simulink model "aircraftControl_smallerStateEKF"  (R2014a)
settings: Solver=ode3  StartTime=0.0  StopTime=50  FixedStep=0.005  RelTol=1e-3
InitFcn:
  | InitialiseModel
values from neighbouring files (symbols this model uses):
  y0 = [0;0;-100;50;0;0;0;x(1);0;0;0;0]    [InitialiseModel.m]
settings Model: Creator=Rudaba  LastModifiedBy=Rudaba
settings DebuggingCC: FcnCallInpInsideContextMsg=EnableAllAsWarning

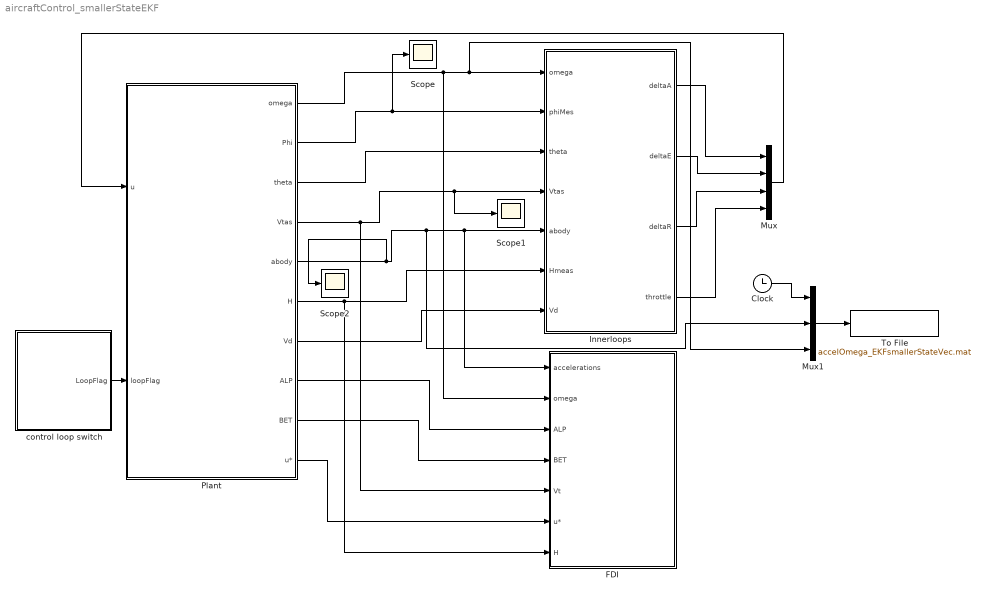
== system aircraftControl_smallerStateEKF ==
  Clock : Clock
  FDI : Subsystem
  Innerloops : Subsystem
  Mux : Mux
  Mux1 : Mux  Inputs=3
  Plant : Subsystem
  Scope : Scope
  Scope1 : Scope
  Scope2 : Scope
      settings: SaveName=ScopeData3
  To File : ToFile  Filename=accelOmega_EKFsmallerStateVec.mat  MatrixName=AO  SaveFormat=Timeseries
  control loop switch : Subsystem
  wires:
  Innerloops/2(deltaE) -> Mux/2
  Innerloops/1(deltaA) -> Mux/1
  Innerloops/3(deltaR) -> Mux/3
  control loop switch/1(LoopFlag) -> Plant/2(loopFlag)
  Innerloops/4(throttle) -> Mux/4
  Mux/1 -> Plant/1(u)
  Plant/1(omega) -> FDI/2(omega), Mux1/3, Innerloops/1(omega)
  Plant/2(Phi) -> Scope/1, Innerloops/2(phiMes)
  Plant/3(theta) -> Innerloops/3(theta)
  Plant/4(Vtas) -> FDI/5(Vt), Scope1/1, Innerloops/4(Vtas)
  Plant/5(abody) -> Scope2/1, Mux1/2, FDI/1(accelerations), Innerloops/5(abody)
  Plant/6(H) -> FDI/7(H), Innerloops/6(Hmeas)
  Plant/7(Vd) -> Innerloops/7(Vd)
  Plant/8(ALP) -> FDI/3(ALP)
  Plant/9(BET) -> FDI/4(BET)
  Plant/10(u*) -> FDI/6(u*)
  Clock/1 -> Mux1/1
  Mux1/1 -> To File/1

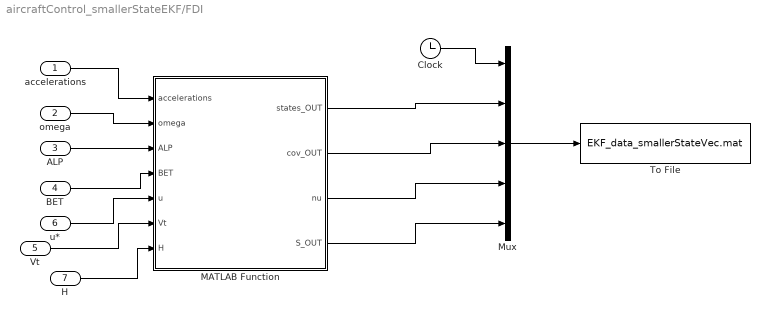
== system aircraftControl_smallerStateEKF/FDI ==
  accelerations : Inport
  omega : Inport  Port=2
  ALP : Inport  Port=3
  BET : Inport  Port=4
  Vt : Inport  Port=5
  u* : Inport  Port=6
  H : Inport  Port=7
  Clock : Clock
  MATLAB Function : MATLAB Function  TreatAsAtomicUnit=on
  Mux : Mux  Inputs=5
  To File : ToFile  Filename=EKF_data_smallerStateVec.mat  MatrixName=EKF  SaveFormat=Timeseries
  wires:
  MATLAB Function/1(states_OUT) -> Mux/2
  MATLAB Function/2(cov_OUT) -> Mux/3
  Mux/1 -> To File/1
  Clock/1 -> Mux/1
  accelerations/1 -> MATLAB Function/1(accelerations)
  omega/1 -> MATLAB Function/2(omega)
  ALP/1 -> MATLAB Function/3(ALP)
  BET/1 -> MATLAB Function/4(BET)
  u*/1 -> MATLAB Function/5(u)
  Vt/1 -> MATLAB Function/6(Vt)
  H/1 -> MATLAB Function/7(H)
  MATLAB Function/3(nu) -> Mux/4
  MATLAB Function/4(S_OUT) -> Mux/5

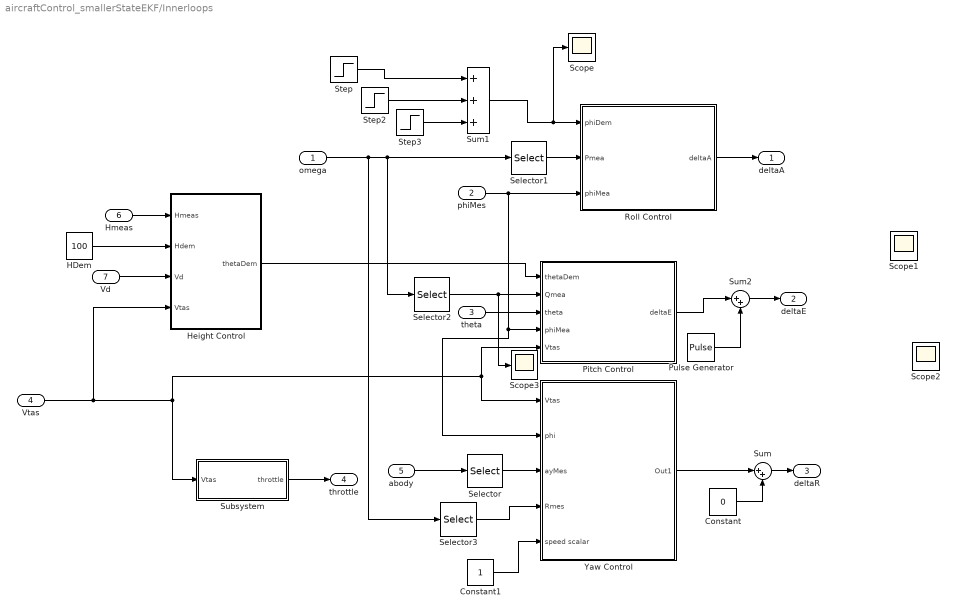
== system aircraftControl_smallerStateEKF/Innerloops ==
  omega : Inport
  phiMes : Inport  Port=2
  theta : Inport  Port=3
  Vtas : Inport  Port=4
  abody : Inport  Port=5
  Hmeas : Inport  Port=6
  Vd : Inport  Port=7
  Constant : Constant  Value=0
  Constant1 : Constant
  HDem : Constant  Value=100
  Height Control : Subsystem
  Pitch Control : Subsystem
  Pulse Generator : DiscretePulseGenerator  PulseType=Time based  Amplitude=0.1  Period=1  PulseWidth=50
  Roll Control : Subsystem
  Scope{,1..3} (4 alike) : Scope
      Scope settings: SaveName=ScopeData2
      Scope1 settings: SaveName=ScopeData11
      Scope2 settings: SaveName=ScopeData12
      Scope3 settings: SaveName=ScopeData13
  Selector : Selector  InputPortWidth=3  Indices=2
  Selector1 : Selector  InputPortWidth=3
  Selector2 : Selector  InputPortWidth=3  Indices=2
  Selector3 : Selector  InputPortWidth=3  Indices=3
  Step : Step  After=0.5  SampleTime=0
  Step2 : Step  Time=40  After=-1  SampleTime=0
  Step3 : Step  Time=70  After=0.5  SampleTime=0
  Subsystem : Subsystem
  Sum : Sum  Inputs=|++
  Sum1 : Sum  Inputs=+++
  Sum2 : Sum  Inputs=|++
  Yaw Control : Subsystem
  deltaA : Outport
  deltaE : Outport  Port=2
  deltaR : Outport  Port=3
  throttle : Outport  Port=4
  wires:
  Height Control/1(thetaDem) -> Pitch Control/1(thetaDem)
  omega/1 -> Selector3/1, Selector1/1, Selector2/1
  phiMes/1 -> Yaw Control/2(phi), Pitch Control/4(phiMea), Roll Control/3(phiMea)
  Selector2/1 -> Scope3/1, Pitch Control/2(Qmea)
  theta/1 -> Pitch Control/3(theta)
  Roll Control/1(deltaA) -> deltaA/1
  Yaw Control/1(Out1) -> Sum/1
  Constant1/1 -> Yaw Control/5(speed scalar)
  abody/1 -> Selector/1
  Selector/1 -> Yaw Control/3(ayMes)
  Constant/1 -> Sum/2
  Sum/1 -> deltaR/1
  Step/1 -> Sum1/1
  Step2/1 -> Sum1/2
  Sum1/1 -> Scope/1, Roll Control/1(phiDem)
  Step3/1 -> Sum1/3
  Hmeas/1 -> Height Control/1(Hmeas)
  HDem/1 -> Height Control/2(Hdem)
  Vd/1 -> Height Control/3(Vd)
  Subsystem/1(throttle) -> throttle/1
  Selector3/1 -> Yaw Control/4(Rmes)
  Vtas/1 -> Height Control/4(Vtas), Subsystem/1(Vtas), Pitch Control/5(Vtas), Yaw Control/1(Vtas)
  Selector1/1 -> Roll Control/2(Pmea)
  Pitch Control/1(deltaE) -> Sum2/1
  Pulse Generator/1 -> Sum2/2
  Sum2/1 -> deltaE/1

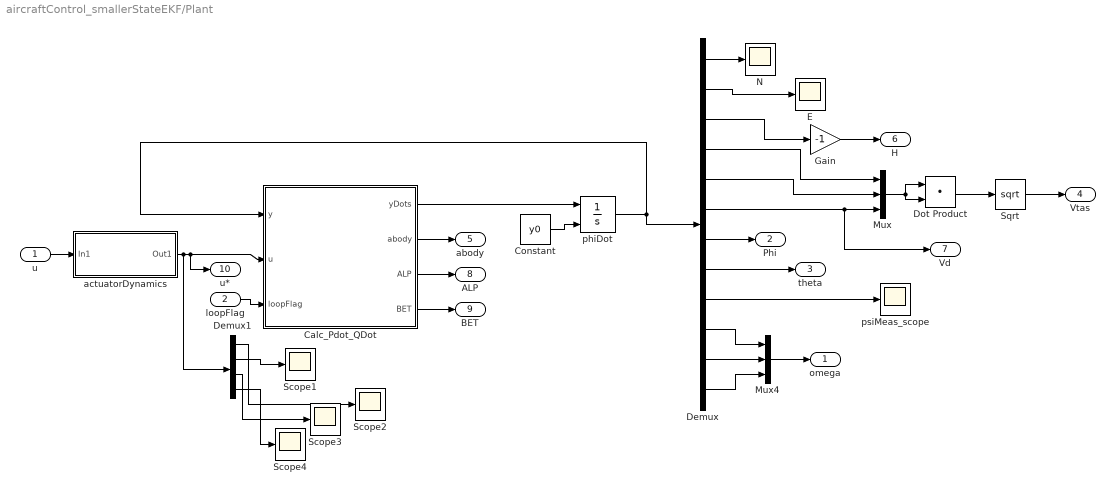
== system aircraftControl_smallerStateEKF/Plant ==
  u : Inport
  loopFlag : Inport  Port=2
  Calc_Pdot_QDot : MATLAB Function  TreatAsAtomicUnit=on
  Constant : Constant  Value=y0
  Demux : Demux  Outputs=12
  Demux1 : Demux
  Dot Product : DotProduct  InputSameDT=on  OutDataTypeStr=Inherit: Inherit via internal rule
  E : Scope
      settings: SaveName=ScopeData8
  Gain : Gain  Gain=-1
  Mux : Mux  Inputs=3
  Mux4 : Mux  Inputs=3
  N : Scope
      settings: SaveName=ScopeData7
  Scope{1..4} (4 alike) : Scope
      Scope1 settings: SaveName=ScopeData4
      Scope2 settings: SaveName=ScopeData6
      Scope3 settings: SaveName=ScopeData9
      Scope4 settings: SaveName=ScopeData10
  Sqrt : Sqrt  SaturateOnIntegerOverflow=on
  actuatorDynamics : Subsystem
  phiDot : Integrator  InitialConditionSource=external
  psiMeas_scope : Scope
      settings: SaveName=ScopeData23
  omega : Outport
  Phi : Outport  Port=2
  theta : Outport  Port=3
  Vtas : Outport  Port=4
  abody : Outport  Port=5
  H : Outport  Port=6
  Vd : Outport  Port=7
  ALP : Outport  Port=8
  BET : Outport  Port=9
  u* : Outport  Port=10
  wires:
  Calc_Pdot_QDot/1(yDots) -> phiDot/1
  Constant/1 -> phiDot/2
  phiDot/1 -> Demux/1, Calc_Pdot_QDot/1(y)
  Demux/7 -> Phi/1
  Demux/8 -> theta/1
  Mux/1 -> Dot Product/2, Dot Product/1
  Dot Product/1 -> Sqrt/1
  Sqrt/1 -> Vtas/1
  Demux/1 -> N/1
  Demux/2 -> E/1
  Demux/4 -> Mux/1
  Demux/5 -> Mux/2
  Demux/6 -> Vd/1, Mux/3
  Demux/9 -> psiMeas_scope/1
  Calc_Pdot_QDot/2(abody) -> abody/1
  actuatorDynamics/1(Out1) -> Demux1/1, u*/1, Calc_Pdot_QDot/2(u)
  u/1 -> actuatorDynamics/1(In1)
  loopFlag/1 -> Calc_Pdot_QDot/3(loopFlag)
  Demux/3 -> Gain/1
  Gain/1 -> H/1
  Calc_Pdot_QDot/3(ALP) -> ALP/1
  Calc_Pdot_QDot/4(BET) -> BET/1
  Demux/10 -> Mux4/1
  Demux/11 -> Mux4/2
  Demux/12 -> Mux4/3
  Mux4/1 -> omega/1
  Demux1/2 -> Scope1/1
  Demux1/1 -> Scope2/1
  Demux1/3 -> Scope3/1
  Demux1/4 -> Scope4/1

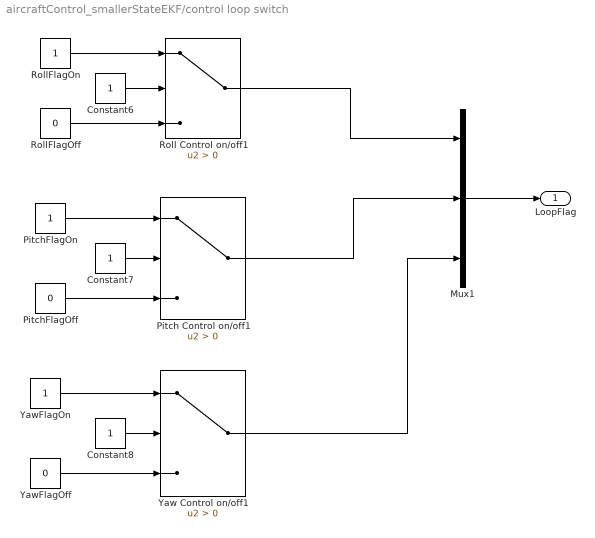
== system aircraftControl_smallerStateEKF/control loop switch ==
  Constant6 : Constant
  Constant7 : Constant
  Constant8 : Constant
  Mux1 : Mux  Inputs=3
  Pitch Control on/off1 : Switch  Criteria=u2 > Threshold
  PitchFlagOff : Constant  Value=0
  PitchFlagOn : Constant
  Roll Control on/off1 : Switch  Criteria=u2 > Threshold
  RollFlagOff : Constant  Value=0
  RollFlagOn : Constant
  Yaw Control on/off1 : Switch  Criteria=u2 > Threshold
  YawFlagOff : Constant  Value=0
  YawFlagOn : Constant
  LoopFlag : Outport
  wires:
  Yaw Control on/off1/1 -> Mux1/3
  Constant6/1 -> Roll Control on/off1/2
  Constant7/1 -> Pitch Control on/off1/2
  Pitch Control on/off1/1 -> Mux1/2
  Roll Control on/off1/1 -> Mux1/1
  Constant8/1 -> Yaw Control on/off1/2
  YawFlagOff/1 -> Yaw Control on/off1/3
  RollFlagOn/1 -> Roll Control on/off1/1
  PitchFlagOn/1 -> Pitch Control on/off1/1
  YawFlagOn/1 -> Yaw Control on/off1/1
  Mux1/1 -> LoopFlag/1
  RollFlagOff/1 -> Roll Control on/off1/3
  PitchFlagOff/1 -> Pitch Control on/off1/3

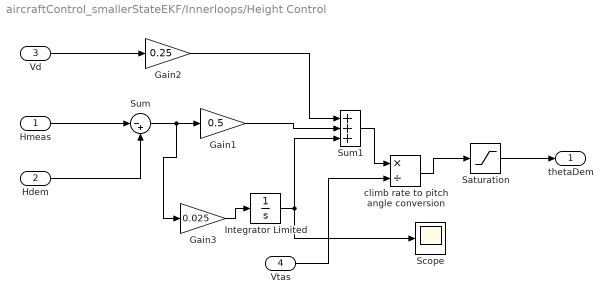
== system aircraftControl_smallerStateEKF/Innerloops/Height Control ==
  Hmeas : Inport
  Hdem : Inport  Port=2
  Vd : Inport  Port=3
  Vtas : Inport  Port=4
  Gain1 : Gain  Gain=0.5
  Gain2 : Gain  Gain=0.25
  Gain3 : Gain  Gain=0.025
  Integrator Limited : Integrator  LimitOutput=on  UpperSaturationLimit=5  LowerSaturationLimit=-5
  Saturation : Saturate  UpperLimit=0.25  LowerLimit=0
  Scope : Scope
      settings: SaveName=ScopeData5  Decimation=10
  Sum : Sum  Inputs=|-+
  Sum1 : Sum  Inputs=+++
  climb rate to pitch angle conversion : Product  Inputs=*/
  thetaDem : Outport
  wires:
  Hdem/1 -> Sum/2
  Hmeas/1 -> Sum/1
  Sum/1 -> Gain3/1, Gain1/1
  Saturation/1 -> thetaDem/1
  Vtas/1 -> climb rate to pitch angle conversion/2
  climb rate to pitch angle conversion/1 -> Saturation/1
  Vd/1 -> Gain2/1
  Gain2/1 -> Sum1/1
  Sum1/1 -> climb rate to pitch angle conversion/1
  Gain1/1 -> Sum1/2
  Integrator Limited/1 -> Sum1/3, Scope/1
  Gain3/1 -> Integrator Limited/1

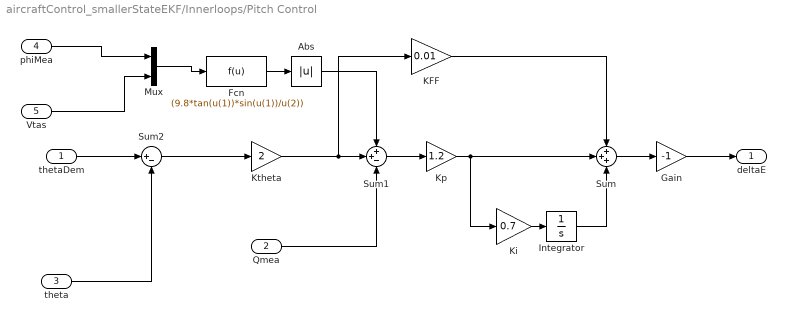
== system aircraftControl_smallerStateEKF/Innerloops/Pitch Control ==
  thetaDem : Inport
  Qmea : Inport  Port=2
  theta : Inport  Port=3
  phiMea : Inport  Port=4
  Vtas : Inport  Port=5
  Abs : Abs
  Fcn : Fcn  Expr=(9.8*tan(u(1))*sin(u(1))/u(2))
  Gain : Gain  Gain=-1
  Integrator : Integrator
  KFF : Gain  Gain=0.01
  Ki : Gain  Gain=0.7
  Kp : Gain  Gain=1.2
  Ktheta : Gain  Gain=2
  Mux : Mux  Inputs=2
  Sum : Sum  Inputs=+++
  Sum1 : Sum  Inputs=++-
  Sum2 : Sum  Inputs=|+-
  deltaE : Outport
  wires:
  Qmea/1 -> Sum1/3
  Sum1/1 -> Kp/1
  Kp/1 -> Ki/1, Sum/2
  KFF/1 -> Sum/1
  Sum/1 -> Gain/1
  Gain/1 -> deltaE/1
  Ktheta/1 -> Sum1/2, KFF/1
  thetaDem/1 -> Sum2/1
  Sum2/1 -> Ktheta/1
  theta/1 -> Sum2/2
  Ki/1 -> Integrator/1
  Vtas/1 -> Mux/2
  Mux/1 -> Fcn/1
  Fcn/1 -> Abs/1
  phiMea/1 -> Mux/1
  Abs/1 -> Sum1/1
  Integrator/1 -> Sum/3

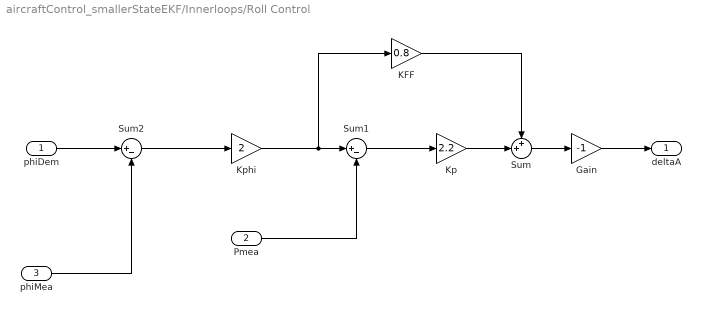
== system aircraftControl_smallerStateEKF/Innerloops/Roll Control ==
  phiDem : Inport
  Pmea : Inport  Port=2
  phiMea : Inport  Port=3
  Gain : Gain  Gain=-1
  KFF : Gain  Gain=0.8
  Kp : Gain  Gain=2.2
  Kphi : Gain  Gain=2
  Sum : Sum  Inputs=++|
  Sum1 : Sum  Inputs=|+-
  Sum2 : Sum  Inputs=|+-
  deltaA : Outport
  wires:
  Pmea/1 -> Sum1/2
  Sum1/1 -> Kp/1
  Kp/1 -> Sum/2
  KFF/1 -> Sum/1
  Sum/1 -> Gain/1
  Gain/1 -> deltaA/1
  Kphi/1 -> KFF/1, Sum1/1
  phiDem/1 -> Sum2/1
  Sum2/1 -> Kphi/1
  phiMea/1 -> Sum2/2

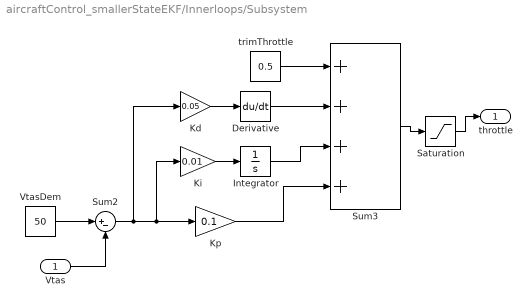
== system aircraftControl_smallerStateEKF/Innerloops/Subsystem ==
  Vtas : Inport
  Derivative : Derivative
  Integrator : Integrator  LimitOutput=on  UpperSaturationLimit=0.5  LowerSaturationLimit=-0.5
  Kd : Gain  Gain=0.05
  Ki : Gain  Gain=0.01
  Kp : Gain  Gain=0.1
  Saturation : Saturate  UpperLimit=1  LowerLimit=0
  Sum2 : Sum  Inputs=|+-
  Sum3 : Sum  Inputs=++++
  VtasDem : Constant  Value=50
  trimThrottle : Constant  Value=0.5
  throttle : Outport
  wires:
  Sum2/1 -> Ki/1, Kp/1, Kd/1
  Kp/1 -> Sum3/4
  trimThrottle/1 -> Sum3/1
  Ki/1 -> Integrator/1
  Integrator/1 -> Sum3/3
  Kd/1 -> Derivative/1
  Derivative/1 -> Sum3/2
  Sum3/1 -> Saturation/1
  Saturation/1 -> throttle/1
  VtasDem/1 -> Sum2/1
  Vtas/1 -> Sum2/2

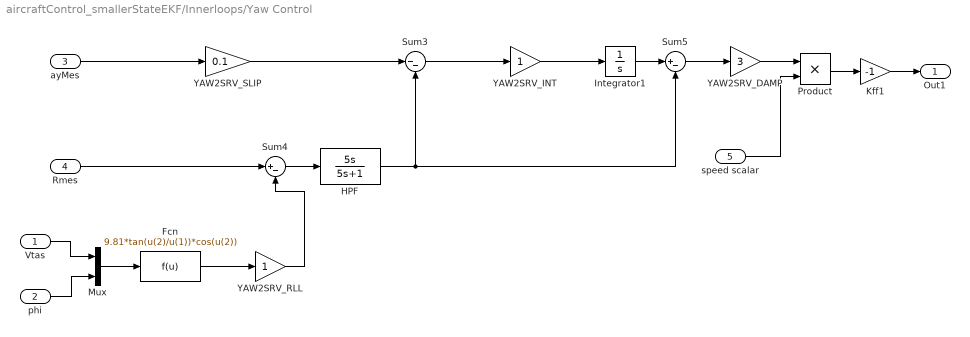
== system aircraftControl_smallerStateEKF/Innerloops/Yaw Control ==
  Vtas : Inport
  phi : Inport  Port=2
  ayMes : Inport  Port=3
  Rmes : Inport  Port=4
  speed scalar : Inport  Port=5
  Fcn : Fcn  Expr=9.81*tan(u(2)/u(1))*cos(u(2))
  HPF : TransferFcn  Numerator=[5 0]  Denominator=[5 1]
  Integrator1 : Integrator  LimitOutput=on  UpperSaturationLimit=0.05  LowerSaturationLimit=-0.05
  Kff1 : Gain  Gain=-1
  Mux : Mux  Inputs=2
  Product : Product
  Sum3 : Sum  Inputs=|--
  Sum4 : Sum  Inputs=|+-
  Sum5 : Sum  Inputs=|+-
  YAW2SRV_DAMP : Gain  Gain=3
  YAW2SRV_INT : Gain
  YAW2SRV_RLL : Gain
  YAW2SRV_SLIP : Gain  Gain=0.1
  Out1 : Outport
  wires:
  Vtas/1 -> Mux/1
  phi/1 -> Mux/2
  Mux/1 -> Fcn/1
  ayMes/1 -> YAW2SRV_SLIP/1
  YAW2SRV_SLIP/1 -> Sum3/1
  Sum3/1 -> YAW2SRV_INT/1
  YAW2SRV_INT/1 -> Integrator1/1
  YAW2SRV_DAMP/1 -> Product/1
  Rmes/1 -> Sum4/1
  Fcn/1 -> YAW2SRV_RLL/1
  Sum4/1 -> HPF/1
  Integrator1/1 -> Sum5/1
  HPF/1 -> Sum3/2, Sum5/2
  Sum5/1 -> YAW2SRV_DAMP/1
  speed scalar/1 -> Product/2
  Product/1 -> Kff1/1
  Kff1/1 -> Out1/1
  YAW2SRV_RLL/1 -> Sum4/2

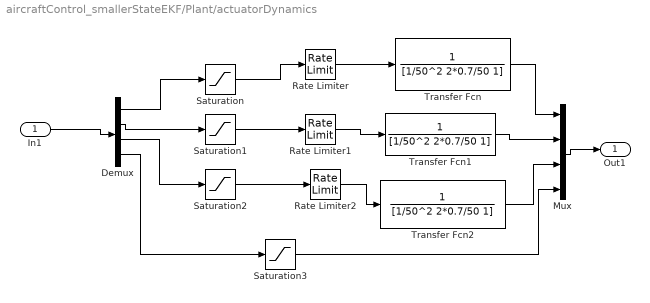
== system aircraftControl_smallerStateEKF/Plant/actuatorDynamics ==
  In1 : Inport
  Demux : Demux
  Mux : Mux
  Rate Limiter : RateLimiter  RisingSlewLimit=5  FallingSlewLimit=-5  SampleTimeMode=inherited
  Rate Limiter1 : RateLimiter  RisingSlewLimit=5  FallingSlewLimit=-5  SampleTimeMode=inherited
  Rate Limiter2 : RateLimiter  RisingSlewLimit=5  FallingSlewLimit=-5  SampleTimeMode=inherited
  Saturation : Saturate  UpperLimit=0.9  LowerLimit=-0.9
  Saturation1 : Saturate  UpperLimit=0.9  LowerLimit=-0.9
  Saturation2 : Saturate  UpperLimit=0.9  LowerLimit=-0.9
  Saturation3 : Saturate  UpperLimit=1  LowerLimit=0
  Transfer Fcn : TransferFcn  Denominator=[1/50^2 2*0.7/50 1]
  Transfer Fcn1 : TransferFcn  Denominator=[1/50^2 2*0.7/50 1]
  Transfer Fcn2 : TransferFcn  Denominator=[1/50^2 2*0.7/50 1]
  Out1 : Outport
  wires:
  In1/1 -> Demux/1
  Mux/1 -> Out1/1
  Demux/1 -> Saturation/1
  Demux/2 -> Saturation1/1
  Demux/3 -> Saturation2/1
  Saturation/1 -> Rate Limiter/1
  Saturation1/1 -> Rate Limiter1/1
  Saturation2/1 -> Rate Limiter2/1
  Rate Limiter/1 -> Transfer Fcn/1
  Transfer Fcn/1 -> Mux/1
  Rate Limiter1/1 -> Transfer Fcn1/1
  Transfer Fcn1/1 -> Mux/2
  Rate Limiter2/1 -> Transfer Fcn2/1
  Transfer Fcn2/1 -> Mux/3
  Demux/4 -> Saturation3/1
  Saturation3/1 -> Mux/4

== matlab function aircraftControl_smallerStateEKF/FDI/MATLAB Function ==
  data: accelerations input; omega input; ALP input; BET input; u input; states_OUT output; Vt input; cov_OUT output; H input; nu output; S_OUT output
function [states_OUT, cov_OUT, nu, S_OUT] = EKF_FDI(accelerations,omega,ALP,BET,u,Vt,H)
%#codegen

[states_OUT, cov_OUT,nu,S_OUT] = simulateEKF_smallerStateVec(accelerations,omega,ALP,BET,u,Vt,H);

== matlab function aircraftControl_smallerStateEKF/Plant/Calc_Pdot_QDot ==
  data: y input; u input; yDots output; abody output; loopFlag input; ALP output; BET output
function [yDots,abody,ALP,BET]  = fcn(y,u,loopFlag)
%#codegen

yDots = zeros(12,1);

%***Constants***
g   = 9.81;
vs  = 340.3;
R2D = 180/pi;
rho = 1.225;%1.225*(1-H/44.331/1000)^4.256;

%***Aircraft Parameters***
S       = 20;
m       = 38924 * 0.453592 / 15;%1905;
b       = 20/3;
cbar    = 3;
Ix      = 24970*14.593903*0.092903/15;
Iy      = 122190*14.593903*0.092903/15;
Iz      = 139800*14.593903*0.092903/15;
Ixz     = 1175*14.593903*0.092903/15;
xCG_ref = 0;
xCG     = 0;

%***Extract data***
N           = y(1);
E           = y(2);
D           = y(3);
vN          = y(4);
vE          = y(5);
vD          = y(6);
phi         = y(7);
theta       = y(8);
psi         = y(9);
p           = y(10);
q           = y(11);
r           = y(12);

H           = -D;

throttle    = u(4);%0.3;%u(1);
deltaA      = u(1);
deltaE      = u(2);
deltaR      = u(3);


%***Calculate Velocities and Angular Velocities***
Cbn         = eul2cbn([phi;theta;psi]);
Cnb         = transpose(Cbn);

wind = zeros(3,1);
vrelN       = vN - wind(1);
vrelE       = vE - wind(2);
vrelD       = vD - wind(3);

Vt          = sqrt(vrelN^2 + vrelE^2 + vrelD^2);

v_body      = Cnb*[vrelN; vrelE; vrelD];

windOmega   = zeros(3,1); 
omegaAero   = [p + windOmega(1); q + windOmega(2); r + windOmega(3)];

%***Calculate Aerodynamic Angles***
alpha       = atan(v_body(3)/v_body(1));%0.05;%atan(v_body(3)/v_body(1));
beta        = asin(v_body(2)/Vt);%0.0;%asin(v_body(2)/Vt);

ALP         = alpha*R2D;
BET         = beta*R2D;
dE          = deltaE*R2D;
dA          = deltaA*R2D;
dR          = deltaR*R2D;


%****Change parameters here for choice of control loop***
if loopFlag(1) == 0
    dA      = 0;
    phidot  = 0;
    pdot    = 0;
end

if loopFlag(2) == 0
    dE          = 0;
    thetadot    = 0;
    qdot        = 0;
end


if loopFlag(3) == 0
    dR = 0;
    psidot = 0;
    rdot   = 0; 
end
%********************************************************

%***Calculate Dynamic Pressure***
qbar = 0.5*rho*Vt^2;

%***Calculate dimensional values***
hT = H/3048;

Tmax = ((30.21-0.668*hT-6.877*hT^2+1.951*hT^3-0.1512*hT^4) + ...
    (Vt/vs).*(-33.8+3.347*hT+18.13*hT^2-5.865*hT^3+0.4757*hT^4) + ...
    (Vt/vs)^2.*(100.8-77.56*hT+5.441*hT^2+2.864*hT^3-0.3355*hT^4) + ...
    (Vt/vs)^3.*(-78.99+101.4*hT-30.28*hT^2+3.236*hT^3-0.1089*hT^4) + ...
    (Vt/vs)^4.*(18.74-31.6*hT+12.04*hT^2-1.785*hT^3+0.09417*hT^4))*4448.22/20; % Newton's

T = Tmax*throttle;

%***Caclulate Aerodynamic Derivatives***
CX = -0.0434 + 2.39e-3*ALP+2.53e-5*BET^2-1.07e-6*ALP*BET^2+9.5e-4*dE-8.5e-7*dE*BET^2+(180*omegaAero(2)*cbar/pi/2/Vt)*(8.73e-3+0.001*ALP-1.75e-4*ALP^2);
CY = -0.012*BET+1.55e-3*dR-8e-6*dR*ALP+(180*b/pi/2/Vt)*(2.25e-3*omegaAero(1)+0.0117*omegaAero(3)-3.67e-4*omegaAero(3)*ALP+1.75e-4*omegaAero(3)*dE);
CZ = -0.131-0.0538*ALP-4.76e-3*dE-3.3e-5*dE*ALP-7.5e-5*dA^2+(180*omegaAero(2)*cbar/pi/2/Vt)*(-0.111+5.17e-3*ALP-1.1e-3*ALP^2);
Cl = -5.98e-4*BET-2.83e-4*ALP*BET+1.51e-5*ALP^2*BET-dA*(6.1e-4+2.5e-5*ALP-2.6e-6*ALP^2)-dR*(-2.3e-4+4.5e-6*ALP)+(180*b/2/pi/Vt)*(-4.12e-3*omegaAero(1)-5.24e-4*omegaAero(1)*ALP+4.36e-5*omegaAero(1)*ALP^2+4.36e-4*omegaAero(3)+1.05e-4*omegaAero(3)*ALP+5.24e-5*omegaAero(3)*dE);
Cm = -6.61e-3-2.67e-3*ALP-6.48e-5*BET^2-2.65e-6*ALP*BET^2-6.54e-3*dE-8.49e-5*dE*ALP+3.74e-6*dE*BET^2-3.5e-5*dA^2+(180*omegaAero(2)*cbar/2/pi/Vt)*(-0.0473-1.57e-3*ALP)+(xCG_ref-xCG)*CZ;
Cn = 2.28e-3*BET+1.79e-6*BET^3+1.4e-5*dA+7.0e-6*dA*ALP-9.0e-4*dR+4.0e-6*dR*ALP+(180*b/2/pi/Vt)*(-6.63e-5*omegaAero(1)-1.92e-5*omegaAero(1)*ALP+5.06e-6*omegaAero(1)*ALP^2-6.06e-3*omegaAero(3)-8.73e-5*omegaAero(3)*dE+8.7e-6*omegaAero(3)*dE*ALP)-cbar/b*(xCG_ref-xCG)*CY;

%***Equations of Motion***
% u = v_body(1);%Vt*cos(alpha)*cos(beta);
% v = v_body(2);%Vt*sin(beta);
% w = v_body(3);%Vt*sin(alpha)*cos(beta);

abody = [(qbar*S*CX+T); qbar*S*CY; qbar*S*CZ]/m;
anav  = Cbn*abody;

vNdot = anav(1);
vEdot = anav(2);
vDdot = g+anav(3);

navAccel = anav + [0;0;g];

% udot = r*v-omegaAero(2)*w-g*sin(theta)+(qbar*S*CX+T)/m;
% vdot = p*w-r*u+g*cos(theta)*sin(phi)+qbar*S*CY/m;
% wdot = q*u-p*v+g*cos(theta)*cos(phi)+qbar*S*CZ/m;

% Vtdot = (u*udot+v*vdot+w*wdot)/Vt;
% alphadot = (u*wdot-w*udot)/(u^2+w^2);
% betadot = (Vt*vdot-v*Vtdot)/Vt^2/sqrt(1-(v/Vt)^2);

c1 = ((Iy-Iz)*Iz-Ixz^2)/(Ix*Iz-Ixz^2);
c2 = (Ix-Iy+Iz)*Ixz/(Ix*Iz-Ixz^2);
c3 = Iz/(Ix*Iz-Ixz^2);
c4 = Ixz/(Ix*Iz-Ixz^2);
c5 = (Iz-Ix)/Iy;
c6 = Ixz/Iy;
c7 = 1/Iy;
c8 = ((Ix-Iy)*Ix-Ixz^2)/(Ix*Iz-Ixz^2);
c9 = Ix/(Ix*Iz-Ixz^2);

heng = 0;
pdot = (c1*r+c2*p+c4*heng)*q+qbar*S*b*(c3*Cl+c4*Cn);
qdot = (c5*p-c7*heng)*r-c6*(p^2-r^2)+qbar*S*cbar*c7*Cm;
rdot = (c8*p-c2*r+c9*heng)*q+qbar*S*b*(c4*Cl+c9*Cn);

% Xdot = u*cos(psi)*cos(theta)+v*(cos(psi)*sin(theta)*sin(phi)-sin(psi)*cos(phi))+w*(cos(psi)*sin(theta)*cos(phi)+sin(psi)*sin(phi));
% Ydot = u*sin(psi)*cos(theta)+v*(sin(psi)*sin(theta)*sin(phi)+cos(psi)*cos(phi))+w*(sin(psi)*sin(theta)*cos(phi)-cos(psi)*sin(phi));
% Ddot = -(u*sin(theta)-v*cos(theta)*sin(phi)-w*cos(theta)*cos(phi));

Ndot = vN;
Edot = vE;
Ddot = vD;

phidot = p+tan(theta)*(q*sin(phi)+r*cos(phi));
thetadot = q*cos(phi)-r*sin(phi);
psidot = (q*sin(phi)+r*cos(phi))/cos(theta);

%****Change parameters here for choice of control loop***
if loopFlag(1) == 0
    dA      = 0;
    phidot  = 0;
    pdot    = 0;
end

if loopFlag(2) == 0
    dE          = 0;
    thetadot    = 0;
    qdot        = 0;
end


if loopFlag(3) == 0
    dR = 0;
    psidot = 0;
    rdot   = 0; 
end
%********************************************************


yDots(1,1) = Ndot;
yDots(2,1) = Edot;
yDots(3,1) = Ddot;
yDots(4,1) = vNdot;
yDots(5,1) = vEdot;
yDots(6,1) = vDdot;
yDots(7,1) = phidot;
yDots(8,1) = thetadot;
yDots(9,1) = psidot;
yDots(10,1) = pdot;
yDots(11,1) = qdot;
yDots(12,1) = rdot;

function Cbn          ... %!< DOUBLE(3,3) the body to navigation frame cosine matrix
          = eul2cbn(  ... %!<
          euler)      ... %!< DOUBLE(3,1) the euler angles (phi, theta, psi) in radians

% DOUBLE cosph sinph costh sinth cosps sinps
cosph = cos(euler(1));
sinph = sin(euler(1));
costh = cos(euler(2));
sinth = sin(euler(2));
cosps = cos(euler(3));
sinps = sin(euler(3));

Cbn =  [costh*cosps, -cosph*sinps + sinph*sinth*cosps, sinph*sinps + cosph*sinth*cosps;
        costh*sinps, cosph*cosps + sinph*sinth*sinps,  -sinph*cosps + cosph*sinth*sinps;
        -sinth       sinph*costh,                      cosph*costh];
